simulink model "DynamicEquation"  (R2017b)
settings: Solver=VariableStepAuto  StartTime=0.0  StopTime=10.0  RelTol=1e-3
undefined symbols (not defined in the file or in its folder): magnitude, Sim_Control
libraries: shared6dof x1, MathLibrary x1
settings Model: Creator=One  LastModifiedBy=One

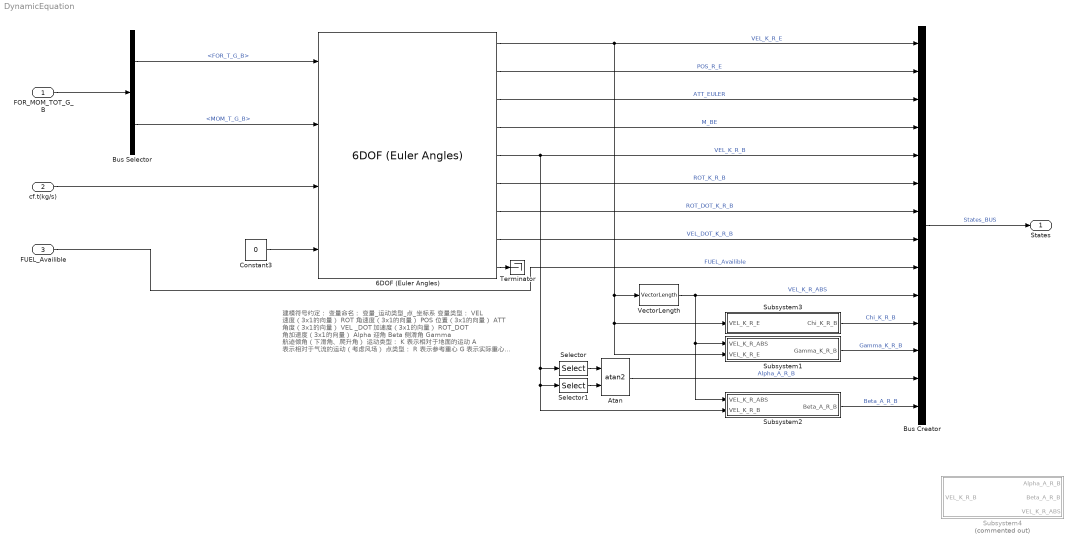
== system DynamicEquation ==
  note: 建模符号约定：
      | 变量命名：
      | 变量_运动类型_点_坐标系
      |
      | 变量类型：
      | VEL 速度（3x1的向量）
      | ROT 角速度（3x1的向量）
      | POS 位置（3x1的向量）
      | ATT 角度（3x1的向量）
      | VEL _DOT 加速度（3x1的向量）
      | ROT_DOT 角加速度（3x1的向量）
      | Alpha 迎角
      | Beta 侧滑角
      | Gamma 航迹倾角（下滑角、爬升角）
      | 运动类型：
      | K 表示相对于地面的运动
      | A 表示相对于气流的运动（考虑风场）
      | 点类型：
      | R 表示参考重心
      | G 表示实际重心
      | 坐标系类型：
      | B 机体系
      | E 地面系 ABS 与坐标系无关，表示该变量的绝对值
  FOR_MOM_TOT_G_B : Inport  OutDataTypeStr=Bus: FOR_MOM_TOT_BUS
  cf.t(kg/s) : Inport  Port=2
  FUEL_Availible : Inport  Port=3
  6DOF (Euler Angles) : shared6dof/6DOF (Euler Angles)  units=Metric (MKS)  mtype=Simple Variable  rep=Euler Angles  xme_0=Sim_Control.init(1,:)  Vm_0=Sim_Control.init(2,:)  eul_0=Sim_Control.init(3,:)  pm_0=Sim_Control.init(4,:)  mass_0=Configuration.Mass  mass_e=Configuration.Mass_Constr  mass_f=Configuration.Mass  inertia=eye(3)  inertia_e=Configuration.Inertia_G_B  inertia_f=Configuration.Inertia_G_B  k_quat=1.0  vre_flag=on  abi_flag=off
      settings: SourceProductBaseCode=AE
  Atan : Trigonometry  Operator=atan2
  Bus Creator : BusCreator  Inputs=14  OutDataTypeStr=Bus: States_BUS
  Bus Selector : BusSelector  OutputSignals=FOR_T_G_B,MOM_T_G_B
  Constant3 : Constant  Value=0
  Selector : Selector  InputPortWidth=3  IndexOptions=Index vector (dialog)  Indices=[3]  OutputSizes=1
  Selector1 : Selector  InputPortWidth=3  IndexOptions=Index vector (dialog)  Indices=[1]  OutputSizes=1
  Subsystem1 : Subsystem
  Subsystem2 : Subsystem
  Subsystem3 : Subsystem
  Subsystem4 : Subsystem  Commented=on
  Terminator : Terminator
  VectorLength : MathLibrary/VectorLength
  States : Outport  OutDataTypeStr=Bus: States_BUS
  wires:
  Constant3/1 -> 6DOF (Euler Angles)/4
  Bus Selector/2 -> 6DOF (Euler Angles)/2  "<MOM_T_G_B>"
  Selector/1 -> Atan/1
  6DOF (Euler Angles)/8 -> Bus Creator/8  "VEL_DOT_K_R_B"
  FUEL_Availible/1 -> Bus Creator/9  "FUEL_Availible"
  cf.t(kg/s)/1 -> 6DOF (Euler Angles)/3
  6DOF (Euler Angles)/9 -> Terminator/1
  6DOF (Euler Angles)/1 -> VectorLength/1, Subsystem3/1(VEL_K_R_E), Subsystem1/2(VEL_K_R_E), Bus Creator/1  "VEL_K_R_E"
  6DOF (Euler Angles)/5 -> Subsystem2/2(VEL_K_R_B), Selector1/1, Selector/1, Bus Creator/5  "VEL_K_R_B"
  6DOF (Euler Angles)/6 -> Bus Creator/6  "ROT_K_R_B"
  FOR_MOM_TOT_G_B/1 -> Bus Selector/1
  Bus Selector/1 -> 6DOF (Euler Angles)/1  "<FOR_T_G_B>"
  Subsystem1/1(Gamma_K_R_B) -> Bus Creator/12  "Gamma_K_R_B"
  Selector1/1 -> Atan/2
  VectorLength/1 -> Subsystem1/1(VEL_K_R_ABS), Subsystem2/1(VEL_K_R_ABS), Bus Creator/10  "VEL_K_R_ABS"
  6DOF (Euler Angles)/4 -> Bus Creator/4  "M_BE"
  Bus Creator/1 -> States/1  "States_BUS"
  6DOF (Euler Angles)/2 -> Bus Creator/2  "POS_R_E"
  Subsystem3/1(Chi_K_R_B) -> Bus Creator/11  "Chi_K_R_B"
  6DOF (Euler Angles)/7 -> Bus Creator/7  "ROT_DOT_K_R_B"
  6DOF (Euler Angles)/3 -> Bus Creator/3  "ATT_EULER"
  Subsystem2/1(Beta_A_R_B) -> Bus Creator/14  "Beta_A_R_B"
  Atan/1 -> Bus Creator/13  "Alpha_A_R_B"

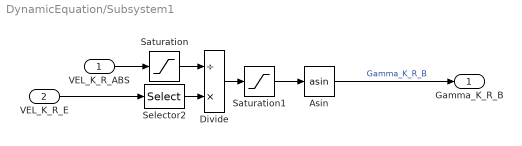
== system DynamicEquation/Subsystem1 ==
  VEL_K_R_ABS : Inport
  VEL_K_R_E : Inport  Port=2
  Asin : Trigonometry  Operator=asin
  Divide : Product  Inputs=/*
  Saturation : Saturate  UpperLimit=inf  LowerLimit=0.01
  Saturation1 : Saturate  UpperLimit=1  LowerLimit=-1
  Selector2 : Selector  InputPortWidth=3  IndexOptions=Index vector (dialog)  Indices=[3]  OutputSizes=1
  Gamma_K_R_B : Outport
  wires:
  Divide/1 -> Saturation1/1
  Asin/1 -> Gamma_K_R_B/1  "Gamma_K_R_B"
  VEL_K_R_E/1 -> Selector2/1
  VEL_K_R_ABS/1 -> Saturation/1
  Selector2/1 -> Divide/2
  Saturation1/1 -> Asin/1
  Saturation/1 -> Divide/1

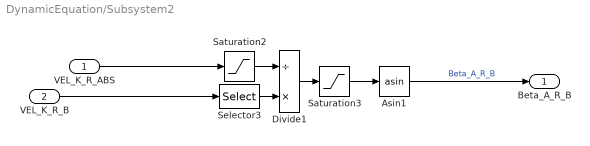
== system DynamicEquation/Subsystem2 ==
  VEL_K_R_ABS : Inport
  VEL_K_R_B : Inport  Port=2
  Asin1 : Trigonometry  Operator=asin
  Divide1 : Product  Inputs=/*
  Saturation2 : Saturate  UpperLimit=inf  LowerLimit=0.01
  Saturation3 : Saturate  UpperLimit=1  LowerLimit=-1
  Selector3 : Selector  InputPortWidth=3  IndexOptions=Index vector (dialog)  Indices=[2]  OutputSizes=1
  Beta_A_R_B : Outport
  wires:
  Saturation2/1 -> Divide1/1
  Asin1/1 -> Beta_A_R_B/1  "Beta_A_R_B"
  Saturation3/1 -> Asin1/1
  Selector3/1 -> Divide1/2
  Divide1/1 -> Saturation3/1
  VEL_K_R_B/1 -> Selector3/1
  VEL_K_R_ABS/1 -> Saturation2/1

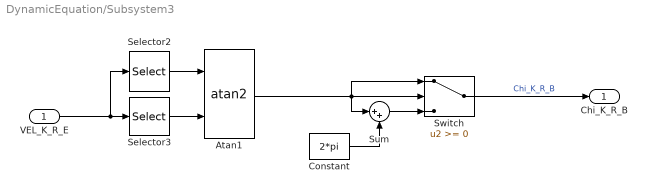
== system DynamicEquation/Subsystem3 ==
  VEL_K_R_E : Inport
  Atan1 : Trigonometry  Operator=atan2
  Constant : Constant  Value=2*pi
  Selector2 : Selector  InputPortWidth=3  IndexOptions=Index vector (dialog)  Indices=[2]  OutputSizes=1
  Selector3 : Selector  InputPortWidth=3  IndexOptions=Index vector (dialog)  Indices=[1]  OutputSizes=1
  Sum : Sum  Inputs=|++
  Switch : Switch
  Chi_K_R_B : Outport
  wires:
  Selector2/1 -> Atan1/1
  Selector3/1 -> Atan1/2
  VEL_K_R_E/1 -> Selector2/1, Selector3/1
  Switch/1 -> Chi_K_R_B/1  "Chi_K_R_B"
  Atan1/1 -> Sum/1, Switch/1, Switch/2
  Constant/1 -> Sum/2
  Sum/1 -> Switch/3

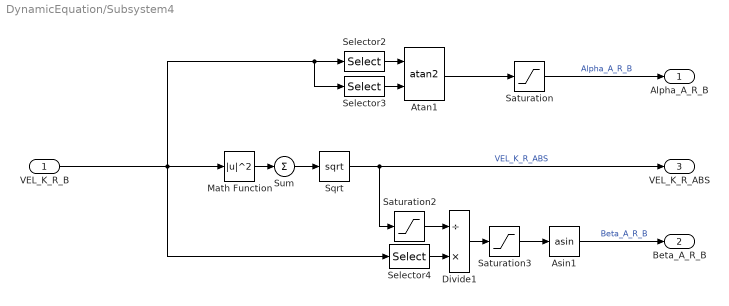
== system DynamicEquation/Subsystem4 ==
  VEL_K_R_B : Inport
  Asin1 : Trigonometry  Operator=asin
  Atan1 : Trigonometry  Operator=atan2
  Divide1 : Product  Inputs=/*
  Math Function : Math  Operator=magnitude^2  SaturateOnIntegerOverflow=on
  Saturation : Saturate  UpperLimit=pi/2  LowerLimit=-pi/2
  Saturation2 : Saturate  UpperLimit=inf  LowerLimit=0.01
  Saturation3 : Saturate  UpperLimit=1  LowerLimit=-11
  Selector2 : Selector  InputPortWidth=3  IndexOptions=Index vector (dialog)  Indices=[3]  OutputSizes=1
  Selector3 : Selector  InputPortWidth=3  IndexOptions=Index vector (dialog)  Indices=[1]  OutputSizes=1
  Selector4 : Selector  InputPortWidth=3  IndexOptions=Index vector (dialog)  Indices=[2]  OutputSizes=1
  Sqrt : Sqrt  SaturateOnIntegerOverflow=on
  Sum : Sum  Inputs=+
  Alpha_A_R_B : Outport
  Beta_A_R_B : Outport  Port=2
  VEL_K_R_ABS : Outport  Port=3
  wires:
  Selector2/1 -> Atan1/1
  Selector3/1 -> Atan1/2
  VEL_K_R_B/1 -> Math Function/1, Selector2/1, Selector3/1, Selector4/1
  Math Function/1 -> Sum/1
  Sum/1 -> Sqrt/1
  Asin1/1 -> Beta_A_R_B/1  "Beta_A_R_B"
  Saturation/1 -> Alpha_A_R_B/1  "Alpha_A_R_B"
  Atan1/1 -> Saturation/1
  Saturation3/1 -> Asin1/1
  Saturation2/1 -> Divide1/1
  Divide1/1 -> Saturation3/1
  Sqrt/1 -> Saturation2/1, VEL_K_R_ABS/1  "VEL_K_R_ABS"
  Selector4/1 -> Divide1/2
